simulink model "dk_truot_r2015a"  (R2015a)
settings: Solver=ode4  SolverMode=SingleTasking  StartTime=0.0  StopTime=30  FixedStep=0.001  RelTol=1e-3
settings Model: CovMetricSettings=dwe  CovHtmlReporting=off  covSaveCumulativeToWorkspaceVar=off  CovSaveSingleToWorkspaceVar=off  CovExternalEMLEnable=on  Creator=ryell  LastModifiedBy=ryell
settings DataIOCC: LimitDataPoints=off  SaveFormat=Dataset
settings DebuggingCC: SFUnexpectedBacktrackingDiag=error  SFNoUnconditionalDefaultTransitionDiag=error
settings HardwareCC: ProdBitPerPointer=64  ProdLargestAtomicFloat=Float  ProdIntDivRoundTo=Zero  ProdEndianess=LittleEndian  ProdHWDeviceType=Specified
settings ModelReferenceCC: PropagateSignalLabelsOutOfModel=on
settings GRTTargetCC: TargetLangStandard=C99 (ISO)  GeneratePreprocessorConditionals=Use local settings

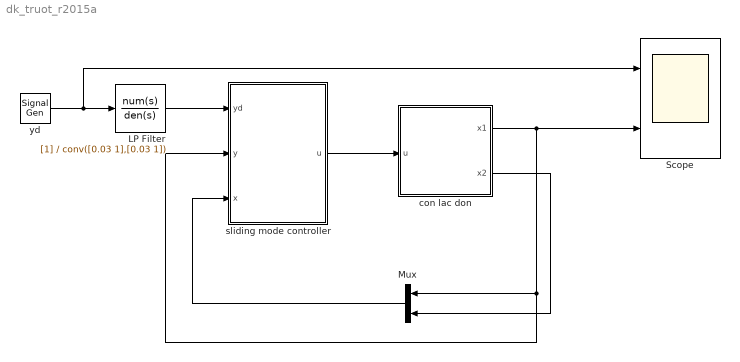
== system dk_truot_r2015a ==
  LP Filter : TransferFcn  Denominator=conv([0.03 1],[0.03 1])
  Mux : Mux  Inputs=2
  Scope : Scope  NumInputPorts=2
      settings: TimeRange=auto  MaxDataPoints=5000  SaveToWorkspace=off  SaveName=ScopeData  YMin=0.51419~-5  YMax=0.53131~5  SampleTime=-1
  con lac don : Subsystem  mask{g=9.81, l=0.2, m=0.5, B=0.05, x1_init=0, x2_init=0}
      mask prompts: g "Gia toc trong truong"; l "Chieu dai thanh treo"; m "Khoi luong vat nang"; B "He so ma sat"; x1_init "Gia tri goc ban dau"; x2_init "Gia tri van toc goc ban dau"
  sliding mode controller : Subsystem  mask{g=9.81, l=0.2, m=0.5, B=0.05, K=100}
      mask prompts: g "Gia toc trong truong"; l "Chieu dai thanh treo"; m "Khoi luong vat nang"; B "He so ma sat"; K "He so mat truot"
  yd : SignalGenerator  WaveForm=square  Amplitude=pi/6  Frequency=0.1
  wires:
  yd/1 -> Scope/1, LP Filter/1
  LP Filter/1 -> sliding mode controller/1(yd)
  sliding mode controller/1(u) -> con lac don/1(u)
  con lac don/1(x1) -> Scope/2, sliding mode controller/2(y), Mux/1
  con lac don/2(x2) -> Mux/2
  Mux/1 -> sliding mode controller/3(x)

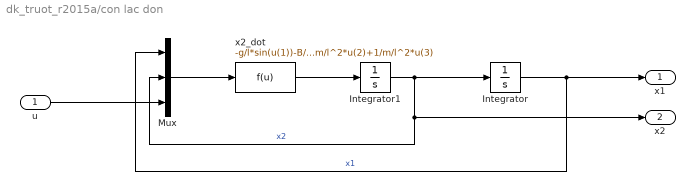
== system dk_truot_r2015a/con lac don ==
  u : Inport
  Integrator : Integrator  InitialCondition=x1_init
  Integrator1 : Integrator  InitialCondition=x2_init
  Mux : Mux  Inputs=3
  x2_dot : Fcn  Expr=-g/l*sin(u(1))-B/m/l^2*u(2)+1/m/l^2*u(3)
  x1 : Outport
  x2 : Outport  Port=2
  wires:
  Integrator1/1 -> x2/1, Mux/2, Integrator/1  "x2"
  u/1 -> Mux/3
  x2_dot/1 -> Integrator1/1
  Integrator/1 -> x1/1, Mux/1  "x1"
  Mux/1 -> x2_dot/1

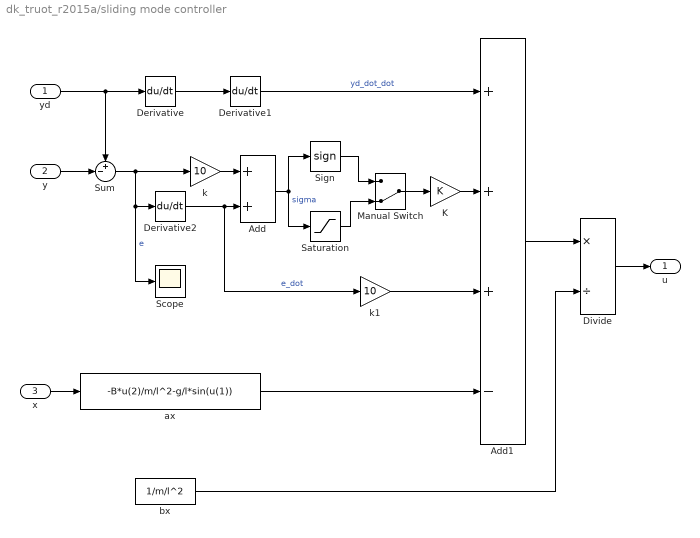
== system dk_truot_r2015a/sliding mode controller ==
  yd : Inport
  y : Inport  Port=2
  x : Inport  Port=3
  Add : Sum
  Add1 : Sum  Inputs=+++-
  Derivative : Derivative
  Derivative1 : Derivative
  Derivative2 : Derivative
  Divide : Product  Inputs=*/
  K : Gain  Gain=K
  Manual Switch : ManualSwitch  CurrentSetting=0
  Saturation : Saturate  UpperLimit=1  LowerLimit=-1
  Scope : Scope
      settings: TimeRange=auto  MaxDataPoints=5000  SaveToWorkspace=off  YMin=-0.3129  YMax=-0.02372  SampleTime=-1
  Sign : Signum
  Sum : Sum  Inputs=+-|
  ax : Fcn  Expr=-B*u(2)/m/l^2-g/l*sin(u(1))
  bx : Constant  Value=1/m/l^2
  k : Gain  Gain=10
  k1 : Gain  Gain=10
  u : Outport
  wires:
  yd/1 -> Sum/1, Derivative/1
  Derivative/1 -> Derivative1/1
  y/1 -> Sum/2
  Sum/1 -> Scope/1, Derivative2/1, k/1  "e"
  Derivative2/1 -> k1/1, Add/2  "e_dot"
  x/1 -> ax/1
  K/1 -> Add1/2
  Derivative1/1 -> Add1/1  "yd_dot_dot"
  ax/1 -> Add1/4
  Add1/1 -> Divide/1
  bx/1 -> Divide/2
  Divide/1 -> u/1
  Manual Switch/1 -> K/1
  Sign/1 -> Manual Switch/1
  Saturation/1 -> Manual Switch/2
  Add/1 -> Saturation/1, Sign/1  "sigma"
  k/1 -> Add/1
  k1/1 -> Add1/3
